simulink model "Projeto_Final_M21"  (R2021a)
settings: Solver=VariableStepAuto  StartTime=0  StopTime=200  FixedStep=0.1  RelTol=1e-3
model workspace (MAT data in the model file):
  N_P0 = 3
  variavelteste = 0
libraries: spsACVoltageSourceLib x1, autolibsharedmappedengines x1, spsCurrentMeasurementLib x1, spsSeriesRLCBranchLib x1, spspowerguiLib x1
(part 1 of 3)
settings Model: EnablePacing=on  Creator=Henrique  LastModifiedBy=Guilherme Moreira

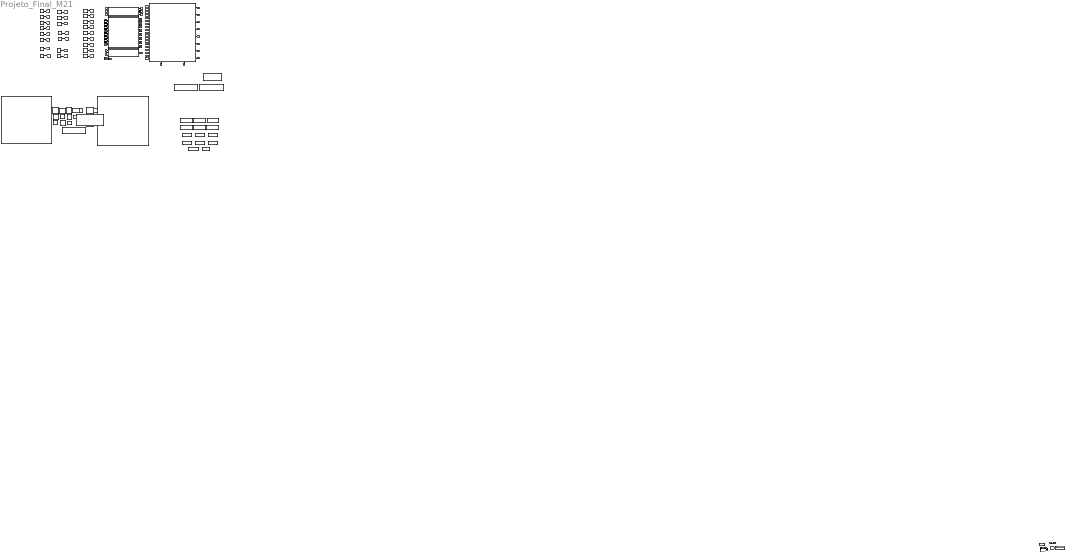
== system Projeto_Final_M21 ==
  note: Pedais Manuais
      |
      |
      |
      |
      |
      |
      |
      |
      |
      |
      |  						Freio												Acelerador
  note: Sistema Start Stop
  note: Transmissão
  note: Motor
  note: Conforto e Segurança
  note: Ar Condicionado
  note: Entradas do Sistema Start/Stop
  note: Subsistemas
  note: Parâmetros Calibráveis
  AC Voltage Source : spsACVoltageSourceLib/AC Voltage Source  Amplitude=100  Phase=0  Frequency=60  SampleTime=0  Measurements=None  BusType=swing  Pref=10e3  Qref=0  Qmin=-inf  Qmax=+inf
  ACELERADOR Slider : CustomTuningWebBlock  LabelPosition=Hide  ShowInitialText=on  Configuration="{\"components\":[{\"name\":\"LinearScaleComponent\",\"settings\":{\"bounds\":{\"max\":1,\"min\":0,\"tickInterval\":\"auto\"},\"internalTickHeightScaleFactor\":0.5,\"labelColor\":[255,255,255],\"labelFont\":{\"font\":\"Arial\",\"fontSize\":12},\"labelTransparency\":1,\"needleImage\":{\"size\":[596,842],\"src\":\"data:image\\/svg+xml;base64,PD94bWwgdmVyc2lvbj0iMS4wIiBlbmNvZGluZz0idXRmLTgiPz4NCjwhLS0gR2VuZXJhdG9yOiBBZG9iZSBJbGx1c3RyYXRvciAyNS4wLjAsIFNWRyBFeHBvcnQgUGx1Zy1JbiAuIFNWRyBWZXJzaW9uOiA2LjAwIEJ1aWxkIDApICAtLT4NCjxzdmcgdmVyc2lvbj0iMS4xIg0KCSBpZD0ic3ZnOCIgeG1sbnM6Y2M9Imh0dHA6Ly9jcmVhdGl2ZWNvbW1vbnMub3JnL25zIyIgeG1sbnM6ZGM9Imh0dHA6Ly9wdXJsLm9yZy9kYy9lbGVtZW50cy8xLjEvIiB4bWxuczppbmtzY2FwZT0iaHR0cDovL3d3dy5pbmtzY2FwZS5vcmcvbmFtZXNw ...(+2420 chars)\",\"srcOrientation\":\"horizontal\"},\"needleOffset\":[-0.8044596912521441,-0.0642123287671233],\"needleSize\":{\"height\":0.4337797619047619,\"width\":0.07668067226890757},\"position\":[0.28322784810126583,0.04399119127516778,0.9196728187919463,0.6087816455696202],\"scaleColors\":[],\"scaleColorsSize\":0.2,\"showLabels\":1,\"showMinorTicks\":0,\"showSpanLine\":1,\"showTicks\":1,\"tickColor\":[234,234,234],\"tickTransparency\":1,\"valueBarColor\":[255,0,0],\"valueBarOffset\":-0.27,\"valueBarSize\":0.1,\"valueBarTransparency\":1}},{\"name\":\"BackgroundImageComponent\",\"settings\":{\"image\":{\"size\":[476,126],\"src\":\"data:image\\/svg+xml;base64,PD94bWwgdmVyc2lvbj0iMS4wIiBlbmNvZGluZz0iVVRGLTgiIHN0YW5kYWxvbmU9Im5vIj8+CjxzdmcKICAgeG1sbnM6ZGM9Imh0dHA6Ly9wdXJsLm9yZy9kYy9lbGVtZW50cy8xLjEvIgogICB4bWxuczpjYz0iaHR0cDovL2NyZWF0aXZlY29tbW9ucy5vcmcvbnMjIgogICB4bWxuczpyZGY9Imh0dHA6Ly93d3cudzMub3JnLzE5OTkvMDIvMjItcmRmLXN5bnRheC1ucyMiCiAgIHhtbG5zOnN2Zz0iaHR0cDovL3d3dy53My5vcmcvMjAwMC9zdmciCiAgIHhtbG5zPSJodHRwOi8vd3d3LnczLm9yZy8yMDAwL3N2ZyIKICAgeG1sbnM6 ...(+2824 chars)\",\"srcOrientation\":\"horizontal\"},\"position\":[0,0,1,1],\"scaleMode\":\"0\"}},{\"name\":\"ForegroundImageComponent\",\"settings\":{\"image\":{\"size\":[0,0],\"src\":\"default\",\"srcOrientation\":[]},\"isForeground\":1,\"position\":[0,0,1,1],\"scaleMode\":\"0\"}}],\"settings\":{\"BindingType\":\"param\",\"aspectRatio\":3.7777777777777777,\"backgroundColor\":[0,0,0,\"1\"],\"backgroundOffset\":0,\"backgroundOpacity\":1,\"fixedAspectRatio\":\"on\",\"foregroundColor\":[252,252,196],\"orientation\":\"horizontal\",\"showBackgroundColor\":false,\"value\":0},\"type\":\"LinearGauge\"}"
  Angulo Direção : Constant  Value=0
  Angulo de Direção : EditField  LabelPosition=Hide  ShowInitialText=on  Alignment=Center
  Battery : LampBlock  LabelPosition=Hide  Icon=Battery
  Capô : SliderSwitchBlock  LabelPosition=Hide
      settings: Values={{'Off', 'On'}, [0 1]}
  Catalyst : LampBlock  LabelPosition=Hide  Icon=Custom  CustomIcon=data:image/svg+xml;base64,PD94bWwgdmVyc2lvbj0iMS4wIiBlbmNvZGluZz0iVVRGLTgiPz4KPHN2ZyB2ZXJzaW9uPSIxLjEiIHhtbG5zPSJodHRwOi8vd3d3LnczLm9yZy8yMDAwL3N2ZyIgd2lkdGg9IjUxMiIgaGVpZ2h0PSI1MTIiPgo8cGF0aCBkPSJNMCAwIEMyLjc2MDU4ODg2IC0wLjAyNTI3NTg4IDUuNTIwNDkzMjUgLTAuMDc4NjA0OTggOC4yODA3MDA2OCAtMC4xMzAwOTY0NCBDMTQuOTU3ODA3OTUgLTAuMjM2OTExNzUgMjEuNjMxMTA3MTQgLTAuMjQxOTI4NDQgMjguMzA4ODM0MzkgLTAuMjA3NDA2MzcgQzMzLjc0NTcxNjQyIC0wLjE4MDcyNzUy ...(+32880 chars)
  Ciclo Direção e Temp Catalisador : Subsystem
  Cinto : SliderSwitchBlock  LabelPosition=Hide
      settings: Values={{'Off', 'On'}, [0 1]}
  Circular Gauge1 : CustomWebBlock  LabelPosition=Hide  ShowInitialText=on  Configuration="{\"components\":[{\"name\":\"CircularScaleComponent\",\"settings\":{\"bounds\":{\"max\":7000,\"min\":0,\"tickInterval\":500},\"direction\":\"cw\",\"flipLimits\":0,\"innerRadius\":0.75,\"internalTickHeightScaleFactor\":1,\"labelColor\":[255,255,200],\"labelFont\":{\"font\":\"Arial\",\"fontSize\":12},\"labelTransparency\":1,\"minorTickHeightScaleFactor\":0.2,\"needleImage\":{\"size\":[200,50],\"src\":\"data:image\\/svg+xml;base64,PD94bWwgdmVyc2lvbj0iMS4wIiBlbmNvZGluZz0idXRmLTgiPz4KPCEtLSBHZW5lcmF0b3I6IEFkb2JlIElsbHVzdHJhdG9yIDI0LjEuMiwgU1ZHIEV4cG9ydCBQbHVnLUluIC4gU1ZHIFZlcnNpb246IDYuMDAgQnVpbGQgMCkgIC0tPgo8c3ZnIHZlcnNpb249IjEuMSIgaWQ9IkxheWVyXzEiIHhtbG5zPSJodHRwOi8vd3d3LnczLm9yZy8yMDAwL3N2ZyIgeG1sbnM6eGxpbms9Imh0dHA6Ly93d3cudzMub3JnLzE5OTkveGxpbmsiIHg9IjBweCIgeT0iMHB4IgoJIHZpZXdCb3g9IjAgMCAyMDAgNTAiIHN0eWxlPSJlbmFibGUtYmFja2dyb3VuZDpuZXcgMCAwIDIwMCA1MDsiIHhtbDpzcGFjZT0icHJlc2VydmUiPgo8c3R5bGUgdHlwZT0idGV4dC9jc3MiPgoJLnN0MHtmaWxsOiNFQzIxMjc7fQo8L3N0eWxlPgo8cGF0aCBjbGFzcz0ic3QwIiBkPSJNMTYyLjgsMTMuN0MxNjksNC40LDE4MS43LDEuOSwxOTEsOC4xczExLjgsMTguOSw1LjYsMjguMnMtMTguOSwxMS44LTI4LjIsNS42bDAsMAoJQzE1OS4xLDM1LjYsMTU2LjYsMjMsMTYyLjgsMTMuN0wxNjIuOCwxMy43eiBNMTY1LjgsMTUuOGMtNS4xLDcuNi0zLjEsMTcuOSw0LjYsMjNjNy42LDUuMSwxNy45LDMuMSwyMy00LjYKCWM1LjEtNy42LDMuMS0xNy45LTQuNi0yM2wwLDBDMTgxLjIsNi4yLDE3MC45LDguMiwxNjUuOCwxNS44eiIvPgo8cGF0aCBjbGFzcz0ic3QwIiBkPSJNMC40LDI1Ljl2LTMuM2wxNTktMi41Yy0wLjcsMi42LTAuNyw1LjIsMCw3LjhMMC40LDI1Ljl6Ii8+CjxjaXJjbGUgY2xhc3M9InN0MCIgY3g9IjE3OS42IiBjeT0iMjQiIHI9IjAuNyIvPgo8L3N2Zz4K\"},\"needleOffset\":[0.18464878250906522,0],\"needleOrientation\":-45,\"needleRotation\":180,\"needleSize\":{\"height\":0.11741692305346914,\"width\":0.46108337545091255},\"outerRadius\":0.9,\"position\":[0.06486742424242424,0.05627705627705628,0.8917748917748918,0.8787878787878788],\"scaleAngle\":270,\"scaleAngleOffset\":135,\"scaleColors\":[{\"color\":[254,51,10],\"max\":7000,\"min\":6000}],\"scaleColorsSize\":0.2,\"scalePosition\":[0,0,1,1],\"showLabels\":1,\"showMinorTicks\":1,\"showSpanLine\":1,\"showTicks\":1,\"tickColor\":[252,252,197],\"tickTransparency\":1,\"valueBarColor\":[0,114,189],\"valueBarPosition\":[0,0,1,1],\"valueBarSize\":0.2,\"valueBarTransparency\":1}},{\"name\":\"BackgroundImageComponent\",\"settings\":{\"image\":{\"size\":[500,500],\"src\":\"data:image\\/svg+xml;base64,PD94bWwgdmVyc2lvbj0iMS4wIiBlbmNvZGluZz0iVVRGLTgiIHN0YW5kYWxvbmU9Im5vIj8+CjxzdmcKICAgeG1sbnM6ZGM9Imh0dHA6Ly9wdXJsLm9yZy9kYy9lbGVtZW50cy8xLjEvIgogICB4bWxuczpjYz0iaHR0cDovL2NyZWF0aXZlY29tbW9ucy5vcmcvbnMjIgogICB4bWxuczpyZGY9Imh0dHA6Ly93d3cudzMub3JnLzE5OTkvMDIvMjItcmRmLXN5bnRheC1ucyMiCiAgIHhtbG5zOnN2Zz0iaHR0cDovL3d3dy53My5vcmcvMjAwMC9zdmciCiAgIHhtbG5zPSJodHRwOi8vd3d3LnczLm9yZy8yMDAwL3N2ZyIKICAgeG1sbnM6 ...(+9964 chars)\"},\"position\":[0,0,1,1],\"scaleMode\":\"0\"}},{\"name\":\"ForegroundImageComponent\",\"settings\":{\"image\":{\"size\":[0,0],\"src\":\"default\",\"srcOrientation\":[]},\"isForeground\":1,\"position\":[0,0,1,1],\"scaleMode\":\"0\"}}],\"settings\":{\"BindingType\":\"signal\",\"aspectRatio\":1.032258064516129,\"backgroundColor\":[0,0,0,\"1\"],\"backgroundOffset\":0.14,\"backgroundOpacity\":1,\"direction\":\"cw\",\"fixedAspectRatio\":\"on\",\"flipLimits\":0,\"orientation\":\"horizontal\",\"showBackgroundColor\":false,\"value\":0},\"type\":\"CircularGauge\"}"
  Circular Gauge2 : CustomWebBlock  LabelPosition=Hide  ShowInitialText=on  Configuration="{\"components\":[{\"name\":\"CircularScaleComponent\",\"settings\":{\"bounds\":{\"max\":75,\"min\":0,\"tickInterval\":\"auto\"},\"direction\":\"cw\",\"flipLimits\":0,\"innerRadius\":0.75,\"internalTickHeightScaleFactor\":1,\"labelColor\":[255,255,200],\"labelFont\":{\"font\":\"Arial\",\"fontSize\":12},\"labelTransparency\":1,\"minorTickHeightScaleFactor\":0.2,\"needleImage\":{\"size\":[200,50],\"src\":\"data:image\\/svg+xml;base64,PD94bWwgdmVyc2lvbj0iMS4wIiBlbmNvZGluZz0idXRmLTgiPz4KPCEtLSBHZW5lcmF0b3I6IEFkb2JlIElsbHVzdHJhdG9yIDI0LjEuMiwgU1ZHIEV4cG9ydCBQbHVnLUluIC4gU1ZHIFZlcnNpb246IDYuMDAgQnVpbGQgMCkgIC0tPgo8c3ZnIHZlcnNpb249IjEuMSIgaWQ9IkxheWVyXzEiIHhtbG5zPSJodHRwOi8vd3d3LnczLm9yZy8yMDAwL3N2ZyIgeG1sbnM6eGxpbms9Imh0dHA6Ly93d3cudzMub3JnLzE5OTkveGxpbmsiIHg9IjBweCIgeT0iMHB4IgoJIHZpZXdCb3g9IjAgMCAyMDAgNTAiIHN0eWxlPSJlbmFibGUtYmFja2dyb3VuZDpuZXcgMCAwIDIwMCA1MDsiIHhtbDpzcGFjZT0icHJlc2VydmUiPgo8c3R5bGUgdHlwZT0idGV4dC9jc3MiPgoJLnN0MHtmaWxsOiNFQzIxMjc7fQo8L3N0eWxlPgo8cGF0aCBjbGFzcz0ic3QwIiBkPSJNMTYyLjgsMTMuN0MxNjksNC40LDE4MS43LDEuOSwxOTEsOC4xczExLjgsMTguOSw1LjYsMjguMnMtMTguOSwxMS44LTI4LjIsNS42bDAsMAoJQzE1OS4xLDM1LjYsMTU2LjYsMjMsMTYyLjgsMTMuN0wxNjIuOCwxMy43eiBNMTY1LjgsMTUuOGMtNS4xLDcuNi0zLjEsMTcuOSw0LjYsMjNjNy42LDUuMSwxNy45LDMuMSwyMy00LjYKCWM1LjEtNy42LDMuMS0xNy45LTQuNi0yM2wwLDBDMTgxLjIsNi4yLDE3MC45LDguMiwxNjUuOCwxNS44eiIvPgo8cGF0aCBjbGFzcz0ic3QwIiBkPSJNMC40LDI1Ljl2LTMuM2wxNTktMi41Yy0wLjcsMi42LTAuNyw1LjIsMCw3LjhMMC40LDI1Ljl6Ii8+CjxjaXJjbGUgY2xhc3M9InN0MCIgY3g9IjE3OS42IiBjeT0iMjQiIHI9IjAuNyIvPgo8L3N2Zz4K\"},\"needleOffset\":[0.18464878250906522,0],\"needleOrientation\":-45,\"needleRotation\":180,\"needleSize\":{\"height\":0.11741692305346914,\"width\":0.46108337545091255},\"outerRadius\":0.9,\"position\":[0.06486742424242424,0.05627705627705628,0.8917748917748918,0.8787878787878788],\"scaleAngle\":270,\"scaleAngleOffset\":135,\"scaleColors\":[],\"scaleColorsSize\":0.2,\"scalePosition\":[0,0,1,1],\"showLabels\":1,\"showMinorTicks\":1,\"showSpanLine\":1,\"showTicks\":1,\"tickColor\":[252,252,197],\"tickTransparency\":1,\"valueBarColor\":[0,114,189],\"valueBarPosition\":[0,0,1,1],\"valueBarSize\":0.2,\"valueBarTransparency\":1}},{\"name\":\"BackgroundImageComponent\",\"settings\":{\"image\":{\"size\":[500,500],\"src\":\"data:image\\/svg+xml;base64,PD94bWwgdmVyc2lvbj0iMS4wIiBlbmNvZGluZz0iVVRGLTgiIHN0YW5kYWxvbmU9Im5vIj8+CjxzdmcKICAgeG1sbnM6ZGM9Imh0dHA6Ly9wdXJsLm9yZy9kYy9lbGVtZW50cy8xLjEvIgogICB4bWxuczpjYz0iaHR0cDovL2NyZWF0aXZlY29tbW9ucy5vcmcvbnMjIgogICB4bWxuczpyZGY9Imh0dHA6Ly93d3cudzMub3JnLzE5OTkvMDIvMjItcmRmLXN5bnRheC1ucyMiCiAgIHhtbG5zOnN2Zz0iaHR0cDovL3d3dy53My5vcmcvMjAwMC9zdmciCiAgIHhtbG5zPSJodHRwOi8vd3d3LnczLm9yZy8yMDAwL3N2ZyIKICAgeG1sbnM6 ...(+9964 chars)\"},\"position\":[0,0,1,1],\"scaleMode\":\"0\"}},{\"name\":\"ForegroundImageComponent\",\"settings\":{\"image\":{\"size\":[0,0],\"src\":\"default\",\"srcOrientation\":[]},\"isForeground\":1,\"position\":[0,0,1,1],\"scaleMode\":\"0\"}}],\"settings\":{\"BindingType\":\"signal\",\"aspectRatio\":1.032258064516129,\"backgroundColor\":[0,0,0,\"1\"],\"backgroundOffset\":0.14,\"backgroundOpacity\":1,\"direction\":\"cw\",\"fixedAspectRatio\":\"on\",\"flipLimits\":0,\"orientation\":\"horizontal\",\"showBackgroundColor\":false,\"value\":0},\"type\":\"CircularGauge\"}"
  Combo Box : ComboBox  LabelPosition=Hide  SelectedLabel=D
      settings: Values={{'P', 'N', 'D', 'R'}, [1 2 3 4]}
  Condições para o Dashboard : MATLAB Function  TreatAsAtomicUnit=on
  Current Measurement : spsCurrentMeasurementLib/Current Measurement  PhasorSimulation=off  OutputType=Complex  PSBequivalent=0
  Delta Ar Condicionado : Constant  Value=2
  Display{,1..10} (11 alike) : Display
  EPB : SliderSwitchBlock  LabelPosition=Hide
      settings: Values={{'Off', 'On'}, [0 1]}
  Engine : LampBlock  LabelPosition=Hide  Icon=Engine
  Engine1 : LampBlock  LabelPosition=Hide  Icon=Custom  CustomIcon=data:image/svg+xml;base64,PD94bWwgdmVyc2lvbj0iMS4wIiBlbmNvZGluZz0iaXNvLTg4NTktMSI/Pg0KPCEtLSBVcGxvYWRlZCB0bzogU1ZHIFJlcG8sIHd3dy5zdmdyZXBvLmNvbSwgR2VuZXJhdG9yOiBTVkcgUmVwbyBNaXhlciBUb29scyAtLT4NCjxzdmcgZmlsbD0iIzAwMDAwMCIgaGVpZ2h0PSI4MDBweCIgd2lkdGg9IjgwMHB4IiB2ZXJzaW9uPSIxLjEiIGlkPSJMYXllcl8xIiB4bWxucz0iaHR0cDovL3d3dy53My5vcmcvMjAwMC9zdmciIHhtbG5zOnhsaW5rPSJodHRwOi8vd3d3LnczLm9yZy8xOTk5L3hsaW5rIiANCgkgdmlld0JveD0iMCAwIDUx ...(+2036 chars)
  Engine2 : LampBlock  LabelPosition=Hide  Icon=Custom  CustomIcon=data:image/svg+xml;base64,PD94bWwgdmVyc2lvbj0iMS4wIiBlbmNvZGluZz0iaXNvLTg4NTktMSI/Pg0KPCEtLSBVcGxvYWRlZCB0bzogU1ZHIFJlcG8sIHd3dy5zdmdyZXBvLmNvbSwgR2VuZXJhdG9yOiBTVkcgUmVwbyBNaXhlciBUb29scyAtLT4NCjxzdmcgZmlsbD0iIzAwMDAwMCIgaGVpZ2h0PSI4MDBweCIgd2lkdGg9IjgwMHB4IiB2ZXJzaW9uPSIxLjEiIGlkPSJDYXBhXzEiIHhtbG5zPSJodHRwOi8vd3d3LnczLm9yZy8yMDAwL3N2ZyIgeG1sbnM6eGxpbms9Imh0dHA6Ly93d3cudzMub3JnLzE5OTkveGxpbmsiIA0KCSB2aWV3Qm94PSIwIDAgNjEy ...(+1612 chars)
  Engine3 : LampBlock  LabelPosition=Hide  Icon=Custom  CustomIcon=data:image/svg+xml;base64,PD94bWwgdmVyc2lvbj0iMS4wIiBlbmNvZGluZz0idXRmLTgiPz4NCjwhLS0gVXBsb2FkZWQgdG86IFNWRyBSZXBvLCB3d3cuc3ZncmVwby5jb20sIEdlbmVyYXRvcjogU1ZHIFJlcG8gTWl4ZXIgVG9vbHMgLS0+DQo8c3ZnIHdpZHRoPSI4MDBweCIgaGVpZ2h0PSI4MDBweCIgdmlld0JveD0iMCAwIDEwMjQgMTAyNCIgZmlsbD0iIzAwMDAwMCIgY2xhc3M9Imljb24iICB2ZXJzaW9uPSIxLjEiIHhtbG5zPSJodHRwOi8vd3d3LnczLm9yZy8yMDAwL3N2ZyI+PHBhdGggZD0iTTM4My4yIDk0MS42Yy00IDAtNi40LTAuOC05LjYtMi40 ...(+3304 chars)
  Engine4 : LampBlock  LabelPosition=Hide  Icon=Custom  CustomIcon=data:image/svg+xml;base64,PD94bWwgdmVyc2lvbj0iMS4wIiBzdGFuZGFsb25lPSJubyI/Pgo8IURPQ1RZUEUgc3ZnIFBVQkxJQyAiLS8vVzNDLy9EVEQgU1ZHIDIwMDEwOTA0Ly9FTiIKICJodHRwOi8vd3d3LnczLm9yZy9UUi8yMDAxL1JFQy1TVkctMjAwMTA5MDQvRFREL3N2ZzEwLmR0ZCI+CjxzdmcgdmVyc2lvbj0iMS4wIiB4bWxucz0iaHR0cDovL3d3dy53My5vcmcvMjAwMC9zdmciCiB3aWR0aD0iMjI4LjAwMDAwMHB0IiBoZWlnaHQ9IjE4Ni4wMDAwMDBwdCIgdmlld0JveD0iMCAwIDIyOC4wMDAwMDAgMTg2LjAwMDAwMCIKIHByZXNlcnZlQXNwZWN0 ...(+2648 chars)
  Engine5 : LampBlock  LabelPosition=Hide  Icon=Custom  CustomIcon=data:image/svg+xml;base64,PD94bWwgdmVyc2lvbj0iMS4wIiBlbmNvZGluZz0iaXNvLTg4NTktMSI/Pg0KPCEtLSBVcGxvYWRlZCB0bzogU1ZHIFJlcG8sIHd3dy5zdmdyZXBvLmNvbSwgR2VuZXJhdG9yOiBTVkcgUmVwbyBNaXhlciBUb29scyAtLT4NCjwhRE9DVFlQRSBzdmcgUFVCTElDICItLy9XM0MvL0RURCBTVkcgMS4xLy9FTiIgImh0dHA6Ly93d3cudzMub3JnL0dyYXBoaWNzL1NWRy8xLjEvRFREL3N2ZzExLmR0ZCI+DQo8c3ZnIGZpbGw9IiMwMDAwMDAiIGhlaWdodD0iODAwcHgiIHdpZHRoPSI4MDBweCIgdmVyc2lvbj0iMS4xIiBpZD0iQ2FwYV8x ...(+1724 chars)
  Engine6 : LampBlock  LabelPosition=Hide  Icon=Custom  CustomIcon=data:image/svg+xml;base64,Cjxzdmcgd2lkdGg9IjEwMCIgaGVpZ2h0PSIxMDAiIHZpZXdCb3g9IjAgMCA2NCA2NCIgeG1sbnM9Imh0dHA6Ly93d3cudzMub3JnLzIwMDAvc3ZnIiBmaWxsPSJub25lIj4KICA8IS0tIElubmVyIGNpcmNsZSB3aXRoIFAgLS0+CiAgPGNpcmNsZSBjeD0iMzIiIGN5PSIzMiIgcj0iMTYiIHN0cm9rZT0iYmxhY2siIHN0cm9rZS13aWR0aD0iMyIvPgogIDx0ZXh0IHg9IjMyIiB5PSIzOCIgZm9udC1mYW1pbHk9IkFyaWFsLCBzYW5zLXNlcmlmIiBmb250LXNpemU9IjE4IiB0ZXh0LWFuY2hvcj0ibWlkZGxlIiBmaWxsPSJibGFjayI+UDwvdGV4dD4KCiAgPCEtLSBMZWZ0IGFyYyAtLT4KICA8cGF0aCBkPSJNMTAgMzJjMC03LjUgMi41LTE0LjUgNy0yMCIgc3Ryb2tlPSJibGFjayIgc3Ryb2tlLXdpZHRoPSIzIiBzdHJva2UtbGluZWNhcD0icm91bmQiLz4KICA8cGF0aCBkPSJNMTAgMzJjMCA3LjUgMi41IDE0LjUgNyAyMCIgc3Ryb2tlPSJibGFjayIgc3Ryb2tlLXdpZHRoPSIzIiBzdHJva2UtbGluZWNhcD0icm91bmQiLz4KCiAgPCEtLSBSaWdodCBhcmMgLS0+CiAgPHBhdGggZD0iTTU0IDMyYzAtNy41LTIuNS0xNC41LTctMjAiIHN0cm9rZT0iYmxhY2siIHN0cm9rZS13aWR0aD0iMyIgc3Ryb2tlLWxpbmVjYXA9InJvdW5kIi8+CiAgPHBhdGggZD0iTTU0IDMyYzAgNy41LTIuNSAxNC41LTcgMjAiIHN0cm9rZT0iYmxhY2siIHN0cm9rZS13aWR0aD0iMyIgc3Ryb2tlLWxpbmVjYXA9InJvdW5kIi8+Cjwvc3ZnPgo=
  Engine7 : LampBlock  LabelPosition=Hide  Icon=Custom  CustomIcon=data:image/svg+xml;base64,PD94bWwgdmVyc2lvbj0iMS4wIiBlbmNvZGluZz0iVVRGLTgiIHN0YW5kYWxvbmU9Im5vIj8+CjwhLS0gVXBsb2FkZWQgdG86IFNWRyBSZXBvLCB3d3cuc3ZncmVwby5jb20sIEdlbmVyYXRvcjogU1ZHIFJlcG8gTWl4ZXIgVG9vbHMgLS0+CjxzdmcgeG1sbnM6ZGM9Imh0dHA6Ly9wdXJsLm9yZy9kYy9lbGVtZW50cy8xLjEvIgogICAgIHhtbG5zOmNjPSJodHRwOi8vY3JlYXRpdmVjb21tb25zLm9yZy9ucyMiCiAgICAgeG1sbnM6cmRmPSJodHRwOi8vd3d3LnczLm9yZy8xOTk5LzAyLzIyLXJkZi1zeW50YXgtbnMjIgogICAgIHht ...(+2684 chars)
  Engine9 : LampBlock  LabelPosition=Hide  Icon=Custom  CustomIcon=data:image/svg+xml;base64,PD94bWwgdmVyc2lvbj0iMS4wIiBlbmNvZGluZz0idXRmLTgiPz4KPCFET0NUWVBFIHN2ZyBQVUJMSUMgIi0vL1czQy8vRFREIFNWRyAxLjAvL0VOIiAiaHR0cDovL3d3dy53My5vcmcvVFIvMjAwMS9SRUMtU1ZHLTIwMDEwOTA0L0RURC9zdmcxMC5kdGQiPgo8c3ZnIHZlcnNpb249IjEuMCIgeG1sbnM9Imh0dHA6Ly93d3cudzMub3JnLzIwMDAvc3ZnIiB3aWR0aD0iMTAyNHB4IiBoZWlnaHQ9IjEwMjRweCIgdmlld0JveD0iMCAwIDEwMjQgMTAyNCIgcHJlc2VydmVBc3BlY3RSYXRpbz0ieE1pZFlNaWQgbWVldCI+CiA8ZyBmaWxs ...(+14896 chars)
  Erro Sistema : Constant  Value=0
  Estado Bateria (SOC) : Constant  Value=80
  Estado da Bateria : EditField  LabelPosition=Hide  ShowInitialText=on  Alignment=Center
  Estado de Carga Bateria : Constant  Value=80
  FREIO Slider : CustomTuningWebBlock  LabelPosition=Hide  ShowInitialText=on  Configuration="{\"components\":[{\"name\":\"LinearScaleComponent\",\"settings\":{\"bounds\":{\"max\":1,\"min\":0,\"tickInterval\":\"auto\"},\"internalTickHeightScaleFactor\":0.5,\"labelColor\":[255,255,255],\"labelFont\":{\"font\":\"Arial\",\"fontSize\":12},\"labelTransparency\":1,\"needleImage\":{\"size\":[596,842],\"src\":\"data:image\\/svg+xml;base64,PD94bWwgdmVyc2lvbj0iMS4wIiBlbmNvZGluZz0idXRmLTgiPz4NCjwhLS0gR2VuZXJhdG9yOiBBZG9iZSBJbGx1c3RyYXRvciAyNS4wLjAsIFNWRyBFeHBvcnQgUGx1Zy1JbiAuIFNWRyBWZXJzaW9uOiA2LjAwIEJ1aWxkIDApICAtLT4NCjxzdmcgdmVyc2lvbj0iMS4xIg0KCSBpZD0ic3ZnOCIgeG1sbnM6Y2M9Imh0dHA6Ly9jcmVhdGl2ZWNvbW1vbnMub3JnL25zIyIgeG1sbnM6ZGM9Imh0dHA6Ly9wdXJsLm9yZy9kYy9lbGVtZW50cy8xLjEvIiB4bWxuczppbmtzY2FwZT0iaHR0cDovL3d3dy5pbmtzY2FwZS5vcmcvbmFtZXNw ...(+2420 chars)\",\"srcOrientation\":\"horizontal\"},\"needleOffset\":[-0.8044596912521441,-0.0642123287671233],\"needleSize\":{\"height\":0.4337797619047619,\"width\":0.07668067226890757},\"position\":[0.2830824088748019,0.04399119127516778,0.9196728187919463,0.6087559429477021],\"scaleColors\":[],\"scaleColorsSize\":0.2,\"showLabels\":1,\"showMinorTicks\":0,\"showSpanLine\":1,\"showTicks\":1,\"tickColor\":[234,234,234],\"tickTransparency\":1,\"valueBarColor\":[255,0,0],\"valueBarOffset\":-0.27,\"valueBarSize\":0.1,\"valueBarTransparency\":1}},{\"name\":\"BackgroundImageComponent\",\"settings\":{\"image\":{\"size\":[476,126],\"src\":\"data:image\\/svg+xml;base64,PD94bWwgdmVyc2lvbj0iMS4wIiBlbmNvZGluZz0iVVRGLTgiIHN0YW5kYWxvbmU9Im5vIj8+CjxzdmcKICAgeG1sbnM6ZGM9Imh0dHA6Ly9wdXJsLm9yZy9kYy9lbGVtZW50cy8xLjEvIgogICB4bWxuczpjYz0iaHR0cDovL2NyZWF0aXZlY29tbW9ucy5vcmcvbnMjIgogICB4bWxuczpyZGY9Imh0dHA6Ly93d3cudzMub3JnLzE5OTkvMDIvMjItcmRmLXN5bnRheC1ucyMiCiAgIHhtbG5zOnN2Zz0iaHR0cDovL3d3dy53My5vcmcvMjAwMC9zdmciCiAgIHhtbG5zPSJodHRwOi8vd3d3LnczLm9yZy8yMDAwL3N2ZyIKICAgeG1sbnM6 ...(+2824 chars)\",\"srcOrientation\":\"horizontal\"},\"position\":[0,0,1,1],\"scaleMode\":\"0\"}},{\"name\":\"ForegroundImageComponent\",\"settings\":{\"image\":{\"size\":[0,0],\"src\":\"default\",\"srcOrientation\":[]},\"isForeground\":1,\"position\":[0,0,1,1],\"scaleMode\":\"0\"}}],\"settings\":{\"BindingType\":\"param\",\"aspectRatio\":3.7721518987341773,\"backgroundColor\":[0,0,0,\"1\"],\"backgroundOffset\":0,\"backgroundOpacity\":1,\"fixedAspectRatio\":\"on\",\"foregroundColor\":[252,252,196],\"orientation\":\"horizontal\",\"showBackgroundColor\":false,\"value\":0},\"type\":\"LinearGauge\"}"
  Gerar Falha : SliderSwitchBlock  LabelPosition=Hide
      settings: Values={{'Off', 'On'}, [0 1]}
  Hill Descent Control : LampBlock  LabelPosition=Hide  Icon=Custom  CustomIcon=data:image/svg+xml;base64,PD94bWwgdmVyc2lvbj0iMS4wIiBlbmNvZGluZz0iaXNvLTg4NTktMSI/Pg0KPCEtLSBVcGxvYWRlZCB0bzogU1ZHIFJlcG8sIHd3dy5zdmdyZXBvLmNvbSwgR2VuZXJhdG9yOiBTVkcgUmVwbyBNaXhlciBUb29scyAtLT4NCjxzdmcgZmlsbD0iIzAwMDAwMCIgdmVyc2lvbj0iMS4xIiBpZD0iTGF5ZXJfMSIgeG1sbnM9Imh0dHA6Ly93d3cudzMub3JnLzIwMDAvc3ZnIiB4bWxuczp4bGluaz0iaHR0cDovL3d3dy53My5vcmcvMTk5OS94bGluayIgDQoJIHZpZXdCb3g9IjAgMCA1MTIgNTEyIiB4bWw6c3BhY2U9InByZXNlcnZlIj4NCjxnPg0KCTxnPg0KCQk8cGF0aCBkPSJNNTA2LjU4Myw5Ljg0N0M1MDEuNzI3LDMuNjM1LDQ5NC4yODYsMCw0ODYuNDAyLDBoLTI1NmMtNi43OTMsMC0xMy4zMDMsMi42OTctMTguMDk5LDcuNTAxbC0yMDQuOCwyMDQuOA0KCQkJYy00LjgwNCw0Ljc5Ni03LjUwMSwxMS4zMDctNy41MDEsMTguMDk5djI1NmMwLDE0LjE0LDExLjQ2LDI1LjYsMjUuNiwyNS42aDQwOS42YzE0LjE0LDAsMjUuNi0xMS40NiwyNS42LTI1LjZWMjMzLjU0OQ0KCQkJbDUwLjQzMi0yMDEuNzQ1QzUxMy4xNDUsMjQuMTU4LDUxMS40MywxNi4wNiw1MDYuNTgzLDkuODQ3eiBNNDM1LjIwMiw0ODYuNGgtNDA5LjZWMjU2aDQwOS42VjQ4Ni40eiBNNDM1LjIwMiwyMzAuNGgtNDA5LjYNCgkJCWwyMDQuOC0yMDQuOGgyNTZMNDM1LjIwMiwyMzAuNHoiLz4NCgk8L2c+DQo8L2c+DQo8Zz4NCgk8Zz4NCgkJPHJlY3QgeD0iMzMyLjgwMiIgeT0iMjgxLjYiIHdpZHRoPSI3Ni44IiBoZWlnaHQ9IjI1LjYiLz4NCgk8L2c+DQo8L2c+DQo8L3N2Zz4=
  Hill Descent Control1 : LampBlock  LabelPosition=Hide  Icon=Custom  CustomIcon=data:image/svg+xml;base64,PHN2ZyB4bWxucz0iaHR0cDovL3d3dy53My5vcmcvMjAwMC9zdmciIHdpZHRoPSIxMDI0IiBoZWlnaHQ9IjEwMjQiIHZpZXdCb3g9IjAgMCAxMDI0IDEwMjQiPgogIDxwYXRoIGQ9Ik0gNzM2IDIwOCBMIDczNSAyMDkgTCA3MzIgMjA5IEwgNzMxIDIxMCBMIDczMCAyMTAgTCA3MjggMjEyIEwgNzI3IDIxMiBMIDcyMyAyMTYgTCA3MjMgMjE3IEwgNjg5IDI1MSBMIDY4OSAyNTIgTCA2ODggMjUzIEwgNjg3IDI1MyBMIDY4MiAyNTggTCA2ODIgMjU5IEwgNjgwIDI2MSBMIDY3OSAyNjEgTCA2NzcgMjYzIEwgNjc3IDI2NCBMIDYwOSAz ...(+20488 chars)
  Hill Descent Control2 : LampBlock  LabelPosition=Hide  Icon=HillDescentControl
  Horizontal Gauge : CustomWebBlock  LabelPosition=Hide  ShowInitialText=on  Configuration="{\"components\":[{\"name\":\"LinearScaleComponent\",\"settings\":{\"bounds\":{\"max\":1,\"min\":0,\"tickInterval\":\"auto\"},\"internalTickHeightScaleFactor\":0.5,\"labelColor\":[255,255,200],\"labelFont\":{\"font\":\"Arial\",\"fontSize\":12},\"labelTransparency\":1,\"needleImage\":{\"size\":[21,75],\"src\":\"data:image\\/svg+xml;base64,PHN2ZyB4bWxucz0iaHR0cDovL3d3dy53My5vcmcvMjAwMC9zdmciIHhtbG5zOnhsaW5rPSJodHRwOi8vd3d3LnczLm9yZy8xOTk5L3hsaW5rIiB2aWV3Qm94PSIwIDAgMjEgNzUiPjxkZWZzPjxzdHlsZT4uY2xzLTF7ZmlsbDpub25lO30uY2xzLTJ7aXNvbGF0aW9uOmlzb2xhdGU7fS5jbHMtM3tjbGlwLXBhdGg6dXJsKCNjbGlwLXBhdGgpO30uY2xzLTR7b3BhY2l0eTowLjM7bWl4LWJsZW5kLW1vZGU6bXVsdGlwbHk7fS5jbHMtNXtmaWxsOiNlYjI2Mjk7fTwvc3R5bGU+PGNsaXBQYXRoIGlkPSJjbGlwLXBhdGgiIHRyYW5zZm9y ...(+1928 chars)\",\"srcOrientation\":\"horizontal\"},\"needleOffset\":[0,0.01094391244870041],\"needleSize\":{\"height\":0.7589285714285714,\"width\":0.11960078534031414},\"position\":[0.06986607142857143,0.01995798319327731,0.9641544117647058,0.8],\"scaleColors\":[],\"scaleColorsSize\":0.2,\"showLabels\":1,\"showMinorTicks\":0,\"showSpanLine\":1,\"showTicks\":1,\"tickColor\":[252,252,197],\"tickTransparency\":1,\"valueBarColor\":[23,89,176],\"valueBarOffset\":0,\"valueBarSize\":0.23,\"valueBarTransparency\":1}},{\"name\":\"BackgroundImageComponent\",\"settings\":{\"image\":{\"size\":[380,101],\"src\":\"data:image\\/svg+xml;base64,PHN2ZyB4bWxucz0iaHR0cDovL3d3dy53My5vcmcvMjAwMC9zdmciIHZpZXdCb3g9IjAgMCAzODAgMTAxIj48ZGVmcz48c3R5bGU+LmNscy0xe2ZpbGw6IzAwMmI0Mjt9LmNscy0ye2ZpbGw6IzQyNzA4Mjt9LmNscy0ze2ZpbGw6IzdjYTBiMjt9PC9zdHlsZT48L2RlZnM+PHRpdGxlPmhvcml6b250YWxfZ2F1Z2VfIGJhY2tncm91bmQ8L3RpdGxlPjxnIGlkPSJMYXllcl8yIiBkYXRhLW5hbWU9IkxheWVyIDIiPjxnIGlkPSJMYXllcl8xLTIiIGRhdGEtbmFtZT0iTGF5ZXIgMSI+PHJlY3QgY2xhc3M9ImNscy0xIiB4PSIxMSIgeT0iMTEiIHdpZHRoPSIzNTgiIGhlaWdodD0iNzkiLz48cGF0aCBjbGFzcz0iY2xzLTIiIGQ9Ik04LDhWOTNIMzcyVjhaTTM2OSw5MEgxMVYxMUgzNjlaIi8+PHBhdGggY2xhc3M9ImNscy0zIiBkPSJNMCwwVjEwMUgzODBWMFpNMzcyLDkzSDhWOEgzNzJaIi8+PC9nPjwvZz48L3N2Zz4=\",\"srcOrientation\":\"horizontal\"},\"position\":[0,0,1,1],\"scaleMode\":\"0\"}},{\"name\":\"ForegroundImageComponent\",\"settings\":{\"image\":{\"size\":[0,0],\"src\":\"default\",\"srcOrientation\":[]},\"isForeground\":1,\"position\":[0,0,1,1],\"scaleMode\":\"0\"}}],\"settings\":{\"BindingType\":\"signal\",\"backgroundColor\":[0,0,0,\"1\"],\"backgroundOffset\":0,\"backgroundOpacity\":1,\"fixedAspectRatio\":\"on\",\"orientation\":\"horizontal\",\"showBackgroundColor\":false,\"value\":0},\"type\":\"LinearGauge\"}"
  Ignição : SliderSwitchBlock  LabelPosition=Hide
      settings: Values={{'Off', 'On'}, [0 1]}
  Ignição Manual : Constant
  Modo de Direção : SliderSwitchBlock  LabelPosition=Hide
      settings: Values={{'Manual', 'Automático'}, [1 0]}
  MultiStateImage : MultiStateImageBlock  LabelPosition=Hide
  MultiStateImage1 : MultiStateImageBlock  LabelPosition=Hide
  MultiStateImage2 : MultiStateImageBlock  LabelPosition=Hide
  Porta : SliderSwitchBlock  LabelPosition=Hide
      settings: Values={{'Off', 'On'}, [0 1]}
  Posição Marcha : Constant  Value=3
  Pressão do Freio : Constant  Value=0.2
  Series RLC Branch : spsSeriesRLCBranchLib/Series RLC Branch  LConnTagsString=__new0  RConnTagsString=__new0  BranchType=RLC  Resistance=1  Inductance=1e-3  SetiL0=off  InitialCurrent=0  Capacitance=1e-6  Setx0=off  InitialVoltage=0  Measurements=None
  Sistema Ar Condicionado : Subsystem
  Start / Stop : Constant
  Start Stop : Subsystem
      settings: PortSchema="{\"entries\":[{\"content\":{\"sides\":[{\"content\":{\"connectorIds\":[\"In1\",\"In2\",\"In3\",\"In4\",\"In5\",\"In6\",\"In7\",\"In8\",\"In9\",\"In10\",\"In11\",\"In12\",\"In13\",\"In14\",\"In15\",\"In16\",\"In17\",\"In18\",\"In19\"]},\"type\":\"ConnectorPlacement.EquallySpacedRectSide\",\"uuid\":\"cae27aae-2f0f-495d-b5de-17320b8abd8f\"},{\"content\":{\"connectorIds\":[\"In20\",\"In21\",\"In22\",\"In23\",\"In24\",\"In25\",\"In26\",\"In27\"],\"side\":\"RIGHT\"},\"type\":\"ConnectorPlacement.EquallySpacedRectSide\",\"uuid\":\"8e8233cc-2459-4a11-817a-071854540998\"},{\"content\":{\"connectorIds\":[],\"side\":\"TOP\"},\"type\":\"ConnectorPlacement.EquallySpacedRectSide\",\"uuid\":\"41c669d9-b680-4e51-b1b6-d6f2b3952c85\"},{\"content\":{\"connectorIds\":[\"Out1\",\"Out2\"],\"side\":\"BOTTOM\"},\"type\":\"ConnectorPlacement.EquallySpacedRectSide\",\"uuid\":\"afe65350-4104-4111-ba67-f67e88854dc7\"}]},\"type\":\"ConnectorPlacement.EquallySpacedConnector\",\"uuid\":\"9a6ef2d3-242d-431b-b81f-5ad437d41931\"}],\"packageUris\":[\"http://schema.mathworks.com/mf0/Connector/R2020b\"],\"version\":\"1.0\"}"
  Start_Stop : SliderSwitchBlock  LabelPosition=Hide
      settings: Values={{'Off', 'On'}, [0 1]}
  Status Capô : Constant
  Status Cinto : Constant
  Status EPB : Constant  Value=0
  Status Inclinacao : EditField  LabelPosition=Hide  ShowInitialText=on  Alignment=Center
  Status Inclinação : Constant  Value=5
  Status Porta : Constant
  Status Transmissão : Constant
  Temp Alvo : EditField  LabelPosition=Hide  ShowInitialText=on  Alignment=Center
  Temp Cabine : EditField  LabelPosition=Hide  ShowInitialText=on  Alignment=Center
  Temp Motor : EditField  LabelPosition=Hide  ShowInitialText=on  Alignment=Center
  Temperatura Alvo : Constant  Value=25
  Temperatura Cabine : Constant  Value=25
  Temperatura Catalisador : Constant  Value=500
  Temperatura Motor : Constant  Value=85
  Temperatura do Motor : Constant  Value=80
  Tempo de Espera : Constant
  Velocidade Veículo Start/Stop : Constant  Value=0
  dt : Subsystem
      settings: PortSchema="{\"entries\":[{\"content\":{\"sides\":[{\"content\":{\"connectorIds\":[]},\"type\":\"ConnectorPlacement.EquallySpacedRectSide\",\"uuid\":\"3aaa574a-b805-45ab-be3e-2ca8cc26472a\"},{\"content\":{\"connectorIds\":[\"Out1\"],\"side\":\"RIGHT\"},\"type\":\"ConnectorPlacement.EquallySpacedRectSide\",\"uuid\":\"d6d6499c-32c1-41e1-9c55-f93729060b31\"},{\"content\":{\"connectorIds\":[\"In1\"],\"side\":\"TOP\"},\"type\":\"ConnectorPlacement.EquallySpacedRectSide\",\"uuid\":\"cf732c2b-fa67-4c40-b189-84cf20c5d0b5\"}]},\"type\":\"ConnectorPlacement.EquallySpacedConnector\",\"uuid\":\"90193743-392a-42ec-b8fa-3aaf5f165a73\"}],\"packageUris\":[\"http://schema.mathworks.com/mf0/Connector/R2020b\"],\"version\":\"1.0\"}"
  powergui : spspowerguiLib/powergui  Priority=1  SimulationMode=Continuous  SampleTime=50e-6  frequency=60  Iterations=50  frequencyindice=60  Pbase=100e6  ErrMax=1e-4  UnitsV=kV  UnitsW=MW  buscounter=0  FunctionMessages=off  echomessages=off  EnableUseOfTLC=off  CurrentSourceSwitches=off  DisableSnubberDevices=off  DisableRonSwitches=off  DisableVfSwitches=off  DisplayEquations=off  AutomaticDiscreteSolvers=off  SolverType=Tustin/Backward Euler (TBE)  Interpol=off  ExternalGateDelay=off  methode=off  Ts=100  x0status=blocks  SPID=on  SwTol=0  HookPort=off  NonlinearTolerance=1e-4  nMaxIteration=100  ContinueOnMaxIteration=off  RestoreLinks=warning  ResistiveCurrentMeasurement=off  Frange=[0:2:500]  Ylog=off  Xlog=on  ShowGrid=off  save=off  variable=ZData  structure=0  ZoomFFT=off  StartTime=0.0  cycles=1  DisplayStyle=1  fundamental=60  FreqAxis=off  MaxFrequency=1000  frequencyindicesteady=1  RmsSteady=1  display=off
  Ângulo de Esterçamento : Constant  Value=90
  Ângulo de Inclinação : Constant  Value=5.7
  wires:
  Start Stop/1(EngineState) -> [EngineState]
  Sistema Ar Condicionado/1(AC_OK) -> [StsArCond]
  [VehicleSpeed] -> Start Stop/1(VehicleSpeed)
  [BrakePressure] -> Start Stop/2(BrakePressure)
  [GearPos] -> Start Stop/7(GearPos)
  Status Cinto/1 -> [StatusCinto]
  Status Capô/1 -> [StCapo]
  Status Porta/1 -> [StPorta]
  Status EPB/1 -> [StEPB]
  Ignição Manual/1 -> [EngineSwitch]
  [THRPressure1] -> Start Stop/3(THRPEDAL)
  [StatusCinto] -> Start Stop/4(SeatBeltStatus)
  [StCapo] -> Start Stop/5(HoodStatus)
  [StPorta] -> Start Stop/6(DoorStatus)
  [StEPB] -> Start Stop/8(EPBStatus)
  [EngineSwitch] -> Start Stop/9(EngineSwitch)
  [CargaBateria] -> Start Stop/11(BattSoc)
  [TempMotor] -> Start Stop/12(EngineTemperature)
  Temperatura Motor/1 -> [TempMotor]
  [StsArCond] -> Start Stop/13(AC_OK)
  [GearPos] -> Ciclo Direção e Temp Catalisador/1(Marcha)
  [EngineSwitch] -> Ciclo Direção e Temp Catalisador/2(EngineSwitch)
  Temperatura Alvo/1 -> [TempTarget]
  Temperatura Cabine/1 -> [TempCabine]
  [TempCabine] -> Sistema Ar Condicionado/1(CabinTemperature)
  [TempTarget] -> Sistema Ar Condicionado/2(TargetTemperature)
  [CatalystTemperature] -> Start Stop/15(CatalystTemperature)
  Angulo Direção/1 -> [SteeringAngle]
  [SteeringAngle] -> Start Stop/14(SteeringAngle)
  Status Inclinação/1 -> [SteepSlope]
  [SteepSlope] -> Start Stop/16(SteepSlope)
  Ciclo Direção e Temp Catalisador/1(CatalystTemperature) -> [CatalystTemperature]
  [StartStop] -> Start Stop/17(StartStopStatus)
  Pressão do Freio/1 -> [BrakePressureVAR]
  Velocidade Veículo Start/Stop/1 -> [VehicleSpeedVAR]
  Temperatura do Motor/1 -> [EngineTemperatureVAR]
  Estado Bateria (SOC)/1 -> [SOC_VAR]
  Temperatura Catalisador/1 -> [CatalystTemperatureVAR]
  Ângulo de Esterçamento/1 -> [SteeringAngleVAR]
  Ângulo de Inclinação/1 -> [SteepSlopeVAR]
  Delta Ar Condicionado/1 -> [DeltaArCondVAR]
  [SteepSlopeVAR] -> Start Stop/20(SteepSlopeVAR)
  [SteeringAngleVAR] -> Start Stop/21(SteeringAngleVAR)
  [CatalystTemperatureVAR] -> Start Stop/22(CatalystTemperatureVAR)
  [SOC_VAR] -> Start Stop/23(SOC_VAR)
  [EngineTemperatureVAR] -> Start Stop/24(EngineTemperatureVAR)
  [VehicleSpeedVAR] -> Start Stop/25(VehicleSpeedVAR)
  [BrakePressureVAR] -> Start Stop/26(BrakePressureVAR)
  [DeltaArCondVAR] -> Sistema Ar Condicionado/3(DeltaArCondVAR)
  Start / Stop/1 -> [StartStop]
  [SteeringAngle] -> Condições para o Dashboard/1(SteeringAngle)
  [SteeringAngleVAR] -> Condições para o Dashboard/2(SteeringAngleVAR)
  [TempMotor] -> Condições para o Dashboard/3(EngineTemperature)
  [EngineTemperatureVAR] -> Condições para o Dashboard/4(EngineTemperatureVAR)
  [CargaBateria] -> Condições para o Dashboard/5(BattSoc)
  [SOC_VAR] -> Condições para o Dashboard/6(SOC_VAR)
  Condições para o Dashboard/1(Dash_Volante) -> Display/1
  Condições para o Dashboard/2(Dash_TempMotor) -> Display1/1
  Condições para o Dashboard/3(Dash_Bat) -> Display2/1
  Condições para o Dashboard/4(Dash_SteepSlope) -> Display3/1
  [SteepSlope] -> Condições para o Dashboard/7(SteepSlope)
  [SteepSlopeVAR] -> Condições para o Dashboard/8(SteepSlopeVAR)
  Tempo de Espera/1 -> [TempoEsperaVAR]
  [TempoEsperaVAR] -> Start Stop/27(TempoEsperaVAR)
  Posição Marcha/1 -> [GearPos]
  Estado de Carga Bateria/1 -> [CargaBateria]
  dt/1(Outport) -> [dt]
  [dt] -> Start Stop/10(dt)
  Status Transmissão/1 -> [StatusDrivetrain]
  [StatusDrivetrain] -> Start Stop/18(StatusDrivetrain)
  Erro Sistema/1 -> [StatusStartStop]
  [StatusStartStop] -> Start Stop/19(autostop_error)
  Start Stop/2(STS) -> [STS]
  Condições para o Dashboard/5(MsgFalha) -> Display4/1
  [StatusStartStop] -> Condições para o Dashboard/9(InputFalha)
  [STS] -> Condições para o Dashboard/10(STS)
  Condições para o Dashboard/6(Dash_Running) -> Display5/1
  Current Measurement/1 -> Display6/1
  Condições para o Dashboard/7(Dash_Catalyst) -> Display7/1
  [CatalystTemperature] -> Condições para o Dashboard/12(CatalystTemp)
  [CatalystTemperatureVAR] -> Condições para o Dashboard/11(CatalystTempVar)
  Condições para o Dashboard/8(Dash_EPB) -> Display8/1
  [StPorta] -> Condições para o Dashboard/14(DoorStatus)
  [StatusCinto] -> Condições para o Dashboard/15(SeatBeltStatus)
  [BrakePressure] -> Condições para o Dashboard/16(BrakePressure)
  [StEPB] -> Condições para o Dashboard/13(EPBStatus)
  [GearPos] -> Condições para o Dashboard/17(GearPos)
  [VehicleSpeed] -> Condições para o Dashboard/18(VehicleSpeed)
  [VehicleSpeed] -> Display9/1
  [EngineState] -> Display10/1
  [EngineState] -> Ciclo Direção e Temp Catalisador/3(EngineState)
  Ciclo Direção e Temp Catalisador/4(rotacao1) -> [rotacao]
  Ciclo Direção e Temp Catalisador/3(BrakePressure1) -> [BrakePressure]
  Ciclo Direção e Temp Catalisador/2(VehicleSpeed1) -> [VehicleSpeed]
  Ciclo Direção e Temp Catalisador/5(THRPressure1) -> [THRPressure1]
  connections:
  AC Voltage Source/LConn1 -- Series RLC Branch/RConn1
  AC Voltage Source/RConn1 -- Current Measurement/LConn1
  Current Measurement/RConn1 -- Series RLC Branch/LConn1
